simulink model "cbuildv0p5"  (R2024b)
settings: Solver=FixedStepAuto  StartTime=0.0  StopTime=12  FixedStep=0.001  RelTol=1e-3
model workspace (MAT data in the model file):
  C = 19480.5566856
  DGain = [16.29965735 16.29965735 15.46224499 15.46224499 15.85491435 21.71073697 22.54158281 11.7271646 11.89023926 12.01707508 12.11854371 12.20156349 12.27074664 12.32928621 12.37946299]
  FBgain = 1
  FFgain = 0.7
  GR = 14.14
  IGain = [117.4799242 117.4799242 87.54143949 87.54143949 65.86609231 58.19090765 57.39102046 195.6414284 195.4270634 195.2603347 195.1269515 195.0178196 194.9268763 194.8499242 194.7839652]
  Izz = 76.97
  Kb = 5
  Kd = 2
  Ki = 10
  Kn = 1
  Kp = 0.1
  L = 1.53
  Mz_to_CMD_TV_delta = 1
  NGain = [2.84450804 2.84450804 4.245826716 5.412937893 3.440885499 2 2 14.58729627 14.58729627 14.58729627 14.58729627 14.58729627 14.58729627 14.58729627 14.58729627]
  PGain = [130.03354 130.03354 132.2979663 135.8088906 130.4448578 122.5111241 121.680406 275.8117795 275.6454267 275.5160406 275.4125314 275.3278419 275.2572671 275.1975499 275.1463636]
  R_e = 0.197
  Tmax = 21
  Tmin = 0
  a = 0.775
  degrees_to_radians = 0.0174772222222
  g = 9.81
  h = 0.225
  kappa_desired = 0.2
  kph_to_m = 0.277777777778
  kph_to_mpers = 0.277777777778
  m = 278
  mu = 1
  rpm_to_radpers = 0.10472
  steering_ratio = 1.17517328292
  t = 1.2
  vx_vector = [0 3.21428571429 6.42857142857 9.64285714286 12.8571428571 16.0714285714 19.2857142857 22.5 25.7142857143 28.9285714286 32.1428571429 35.3571428571 38.5714285714 41.7857142857 45]
libraries: slpidlib x2, Solver_SF x1, simulink x1
settings Model: Creator=kara.28  LastModifiedBy=kara.28

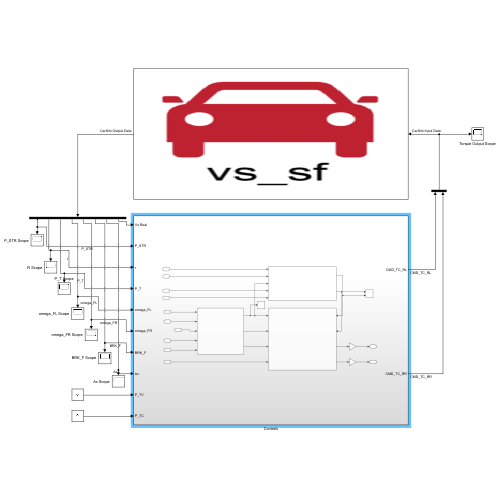
[thumbnail: Simulink's stored preview of the top-level diagram]
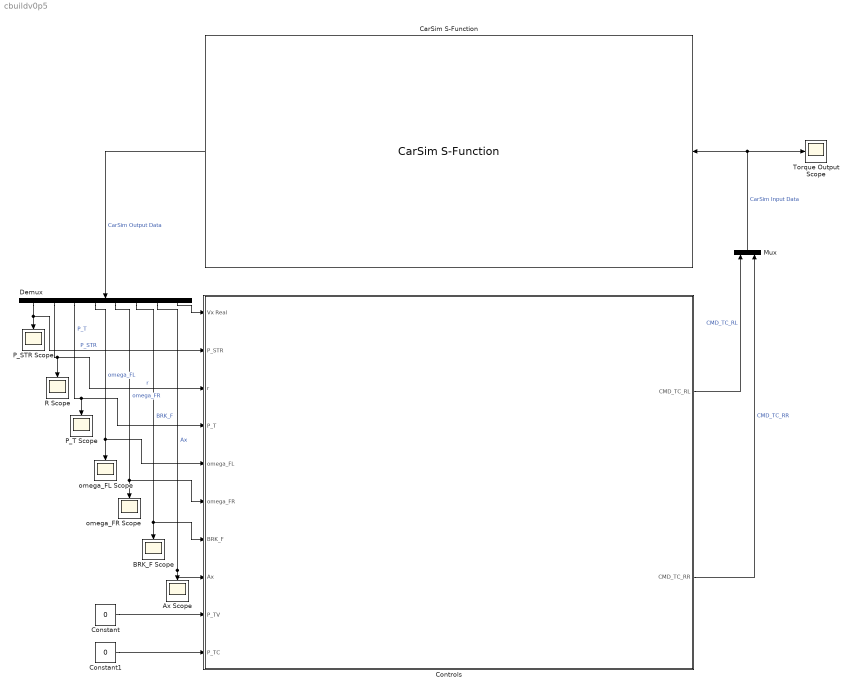
== system cbuildv0p5 ==
  Ax Scope : Scope
  BRK_F Scope : Scope
  CarSim S-Function : Solver_SF/CarSim S-Function  Priority=1  SIMFILE=simfile.sim  Run_RTs=off  vs_state_ind=Run  StopMode_ind=Vehicle Model
  Constant : Constant  Value=0
  Constant1 : Constant  Value=0
  Controls : Subsystem
  Demux : Demux  Outputs=8
  Mux : Mux  Inputs=2
  P_STR Scope : Scope
  P_T Scope : Scope
  R Scope : Scope
  Torque Output Scope : Scope
  omega_FL Scope : Scope
  omega_FR Scope : Scope
  wires:
  Constant/1 -> Controls/9(P_TV)
  Constant1/1 -> Controls/10(P_TC)
  Mux/1 -> Torque Output Scope/1, CarSim S-Function/1  "CarSim Input Data"
  CarSim S-Function/1 -> Demux/1  "CarSim Output Data"
  Demux/1 -> P_STR Scope/1, Controls/2(P_STR)  "P_STR"
  Demux/2 -> R Scope/1, Controls/3(r)  "r"
  Demux/3 -> P_T Scope/1, Controls/4(P_T)  "P_T"
  Demux/4 -> omega_FL Scope/1, Controls/5(omega_FL)  "omega_FL"
  Demux/5 -> omega_FR Scope/1, Controls/6(omega_FR)  "omega_FR"
  Demux/6 -> BRK_F Scope/1, Controls/7(BRK_F)  "BRK_F"
  Demux/7 -> Ax Scope/1, Controls/8(Ax)  "Ax"
  Controls/1(CMD_TC_RL) -> Mux/1  "CMD_TC_RL"
  Controls/2(CMD_TC_RR) -> Mux/2  "CMD_TC_RR"
  Demux/8 -> Controls/1(Vx Real)

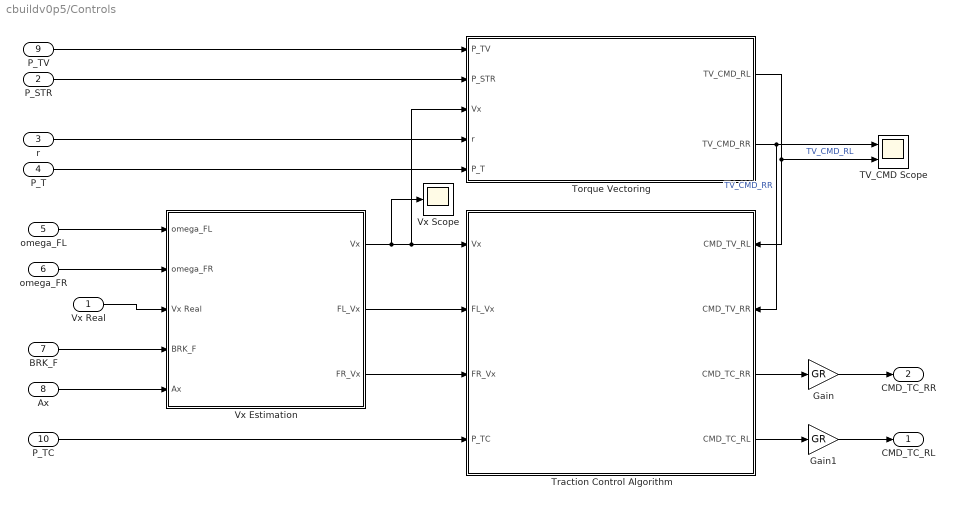
== system cbuildv0p5/Controls ==
  Vx Real : Inport
  P_STR : Inport  Port=2
  r : Inport  Port=3
  P_T : Inport  Port=4
  omega_FL : Inport  Port=5
  omega_FR : Inport  Port=6
  BRK_F : Inport  Port=7
  Ax : Inport  Port=8
  P_TV : Inport  Port=9
  P_TC : Inport  Port=10
  Gain : Gain  Gain=GR
  Gain1 : Gain  Gain=GR
  TV_CMD Scope : Scope  NumInputPorts=2
  Torque Vectoring : Subsystem
  Traction Control Algorithm : Subsystem
      settings: PortSchema="{\"entries\":[{\"content\":{\"sides\":[{\"content\":{\"connectorIds\":[\"In1\",\"In2\",\"In3\",\"In4\"]},\"type\":\"ConnectorPlacement.EquallySpacedRectSide\",\"uuid\":\"6d3224cc-3493-4876-87bf-cb750c54d205\"},{\"content\":{\"connectorIds\":[\"In5\",\"In6\",\"Out1\",\"Out2\"],\"side\":\"RIGHT\"},\"type\":\"ConnectorPlacement.EquallySpacedRectSide\",\"uuid\":\"16bb671c-e18d-4977-8b66-2f7bbb636356\"},{\"content\":{\"side\":\"TOP\"},\"type\":\"ConnectorPlacement.EquallySpacedRectSide\",\"uuid\":\"70c91239-ad82-48f3-8aa3-48d7bdfb7bbb\"}]},\"type\":\"ConnectorPlacement.EquallySpacedConnector\",\"uuid\":\"0f8ba5f7-72f2-430e-8458-63f00911aa7a\"}],\"packageUris\":[\"http://schema.mathworks.com/mf0/Connector/R2020b\"],\"version\":\"1.0\"}"
  Vx Estimation : Subsystem
  Vx Scope : Scope
  CMD_TC_RL : Outport
  CMD_TC_RR : Outport  Port=2
  wires:
  omega_FL/1 -> Vx Estimation/1(omega_FL)
  Vx Estimation/3(FR_Vx) -> Traction Control Algorithm/3(FR_Vx)
  Torque Vectoring/1(TV_CMD_RL) -> Traction Control Algorithm/5(CMD_TV_RL), TV_CMD Scope/2  "TV_CMD_RL"
  P_STR/1 -> Torque Vectoring/2(P_STR)
  Vx Estimation/2(FL_Vx) -> Traction Control Algorithm/2(FL_Vx)
  Vx Estimation/1(Vx) -> Vx Scope/1, Torque Vectoring/3(Vx), Traction Control Algorithm/1(Vx)
  P_T/1 -> Torque Vectoring/5(P_T)
  Ax/1 -> Vx Estimation/5(Ax)
  BRK_F/1 -> Vx Estimation/4(BRK_F)
  P_TC/1 -> Traction Control Algorithm/4(P_TC)
  omega_FR/1 -> Vx Estimation/2(omega_FR)
  Traction Control Algorithm/2(CMD_TC_RL) -> Gain1/1
  P_TV/1 -> Torque Vectoring/1(P_TV)
  Traction Control Algorithm/1(CMD_TC_RR) -> Gain/1
  r/1 -> Torque Vectoring/4(r)
  Torque Vectoring/2(TV_CMD_RR) -> Traction Control Algorithm/6(CMD_TV_RR), TV_CMD Scope/1  "TV_CMD_RR"
  Vx Real/1 -> Vx Estimation/3(Vx Real)
  Gain/1 -> CMD_TC_RR/1
  Gain1/1 -> CMD_TC_RL/1

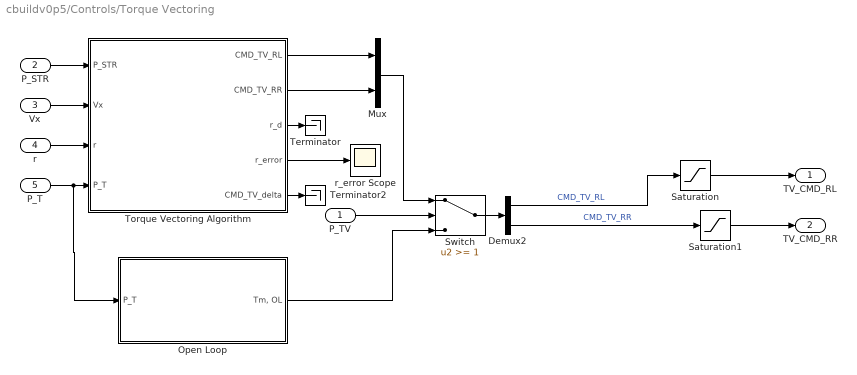
== system cbuildv0p5/Controls/Torque Vectoring ==
  P_TV : Inport
  P_STR : Inport  Port=2
  Vx : Inport  Port=3
  r : Inport  Port=4
  P_T : Inport  Port=5
  Demux2 : Demux  Outputs=2
  Mux : Mux  Inputs=2
  Open Loop : Subsystem
  Saturation : Saturate  UpperLimit=Tmax  LowerLimit=Tmin
  Saturation1 : Saturate  UpperLimit=Tmax  LowerLimit=Tmin
  Switch : Switch  Threshold=1  SaturateOnIntegerOverflow=off  InputSameDT=off
  Terminator : Terminator
  Terminator2 : Terminator
  Torque Vectoring Algorithm : Subsystem
  r_error Scope : Scope
  TV_CMD_RL : Outport
  TV_CMD_RR : Outport  Port=2
  wires:
  Demux2/2 -> Saturation1/1  "CMD_TV_RR"
  Mux/1 -> Switch/1
  P_TV/1 -> Switch/2
  Torque Vectoring Algorithm/2(CMD_TV_RR) -> Mux/2
  Demux2/1 -> Saturation/1  "CMD_TV_RL"
  Open Loop/1("Tm, OL") -> Switch/3
  Torque Vectoring Algorithm/1(CMD_TV_RL) -> Mux/1
  Switch/1 -> Demux2/1
  P_STR/1 -> Torque Vectoring Algorithm/1(P_STR)
  Vx/1 -> Torque Vectoring Algorithm/2(Vx)
  r/1 -> Torque Vectoring Algorithm/3(r)
  P_T/1 -> Open Loop/1(P_T), Torque Vectoring Algorithm/4(P_T)
  Torque Vectoring Algorithm/3(r_d) -> Terminator/1
  Torque Vectoring Algorithm/4(r_error) -> r_error Scope/1
  Torque Vectoring Algorithm/5(CMD_TV_delta) -> Terminator2/1
  Saturation/1 -> TV_CMD_RL/1
  Saturation1/1 -> TV_CMD_RR/1

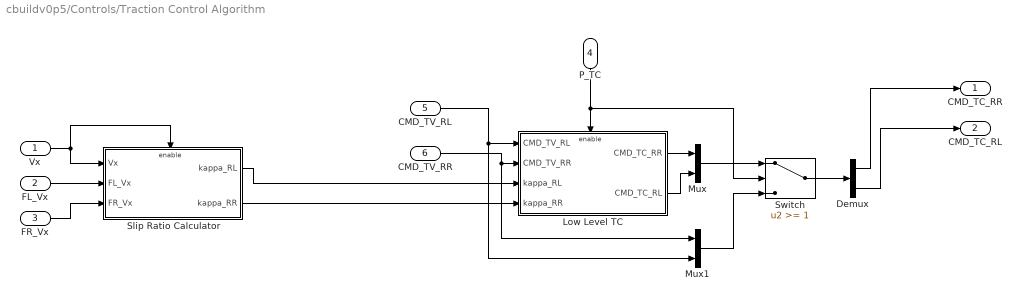
== system cbuildv0p5/Controls/Traction Control Algorithm ==
  Vx : Inport
  FL_Vx : Inport  Port=2
  FR_Vx : Inport  Port=3
  P_TC : Inport  Port=4
  CMD_TV_RL : Inport  Port=5
  CMD_TV_RR : Inport  Port=6
  Demux : Demux  Outputs=2
  Low Level TC : Subsystem
  Mux : Mux  Inputs=2
  Mux1 : Mux  Inputs=2
  Slip Ratio Calculator : Subsystem
  Switch : Switch  Threshold=1  SaturateOnIntegerOverflow=off  InputSameDT=off
  CMD_TC_RR : Outport
  CMD_TC_RL : Outport  Port=2
  wires:
  Slip Ratio Calculator/2(kappa_RR) -> Low Level TC/4(kappa_RR)
  Slip Ratio Calculator/1(kappa_RL) -> Low Level TC/3(kappa_RL)
  FL_Vx/1 -> Slip Ratio Calculator/2(FL_Vx)
  Vx/1 -> Slip Ratio Calculator/Enable, Slip Ratio Calculator/1(Vx)
  FR_Vx/1 -> Slip Ratio Calculator/3(FR_Vx)
  CMD_TV_RL/1 -> Mux1/2, Low Level TC/1(CMD_TV_RL)
  CMD_TV_RR/1 -> Mux1/1, Low Level TC/2(CMD_TV_RR)
  Low Level TC/1(CMD_TC_RR) -> Mux/1
  Low Level TC/2(CMD_TC_RL) -> Mux/2
  Mux/1 -> Switch/1
  Mux1/1 -> Switch/3
  Switch/1 -> Demux/1
  Demux/1 -> CMD_TC_RR/1
  Demux/2 -> CMD_TC_RL/1
  P_TC/1 -> Switch/2, Low Level TC/Enable

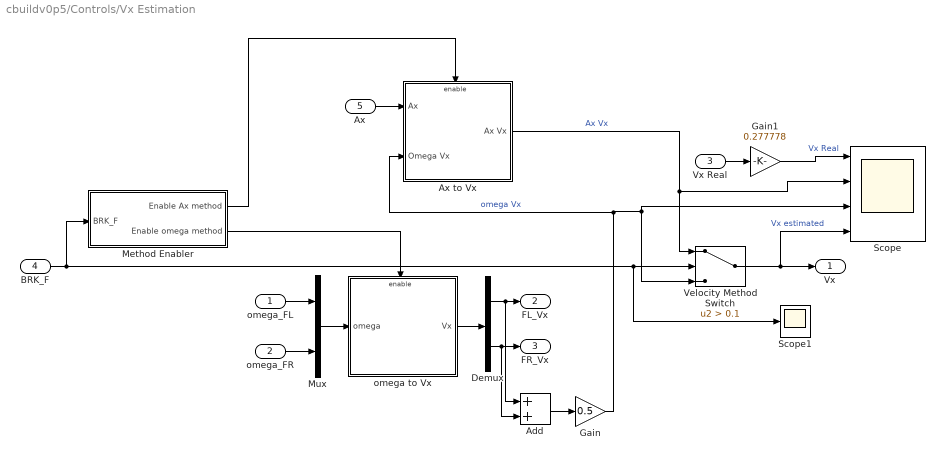
== system cbuildv0p5/Controls/Vx Estimation ==
  omega_FL : Inport
  omega_FR : Inport  Port=2
  Vx Real : Inport  Port=3
  BRK_F : Inport  Port=4
  Ax : Inport  Port=5
  Add : Sum
  Ax to Vx : Subsystem
  Demux : Demux  Outputs=2
  Gain : Gain  Gain=0.5
  Gain1 : Gain  Gain=0.277778
  Method Enabler : Subsystem
  Mux : Mux  Inputs=2
  Scope : Scope  NumInputPorts=4
  Scope1 : Scope
  Velocity Method Switch : Switch  Criteria=u2 > Threshold  Threshold=0.1  SaturateOnIntegerOverflow=off  InputSameDT=off
  omega to Vx : Subsystem
  Vx : Outport
  FL_Vx : Outport  Port=2
  FR_Vx : Outport  Port=3
  wires:
  Mux/1 -> omega to Vx/1(omega)
  omega to Vx/1(Vx) -> Demux/1
  Demux/2 -> Add/2, FR_Vx/1
  omega_FR/1 -> Mux/2
  omega_FL/1 -> Mux/1
  Demux/1 -> Add/1, FL_Vx/1
  BRK_F/1 -> Scope1/1, Velocity Method Switch/2, Method Enabler/1(BRK_F)
  Add/1 -> Gain/1
  Gain/1 -> Velocity Method Switch/3, Scope/3, Ax to Vx/2(Omega Vx)  "omega Vx"
  Velocity Method Switch/1 -> Vx/1, Scope/4  "Vx estimated"
  Ax/1 -> Ax to Vx/1(Ax)
  Ax to Vx/1(Ax Vx) -> Velocity Method Switch/1, Scope/2  "Ax Vx"
  Method Enabler/2(Enable omega method) -> omega to Vx/Enable
  Vx Real/1 -> Gain1/1
  Gain1/1 -> Scope/1  "Vx Real"
  Method Enabler/1(Enable Ax method) -> Ax to Vx/Enable

== system cbuildv0p5/Controls/Torque Vectoring/Open Loop ==
  P_T : Inport
  Gain : Gain  Gain=Tmax
  "Tm, OL" : Outport
  wires:
  P_T/1 -> Gain/1
  Gain/1 -> "Tm, OL"/1

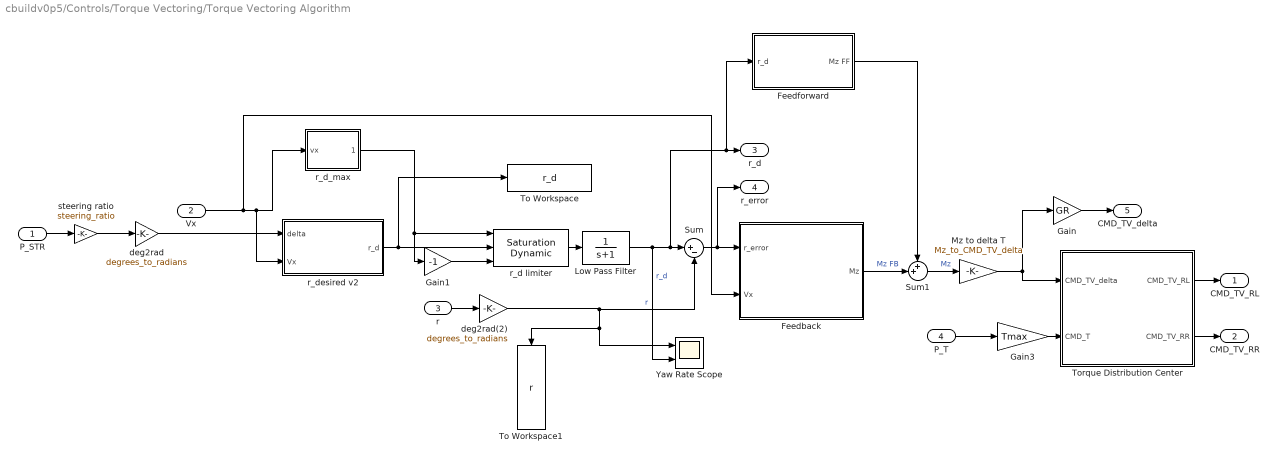
== system cbuildv0p5/Controls/Torque Vectoring/Torque Vectoring Algorithm ==
  P_STR : Inport
  Vx : Inport  Port=2
  r : Inport  Port=3
  P_T : Inport  Port=4
  Feedback : Subsystem
  Feedforward : Subsystem
  Gain : Gain  Gain=GR
  Gain1 : Gain  Gain=-1
  Gain3 : Gain  Gain=Tmax
  Low Pass Filter : TransferFcn  Denominator=[1 1]
  Mz to delta T : Gain  Gain=Mz_to_CMD_TV_delta
  Sum : Sum  Inputs=|+-
  Sum1 : Sum  Inputs=++|
  To Workspace : ToWorkspace  VariableName=r_d  SampleTime=-1
  To Workspace1 : ToWorkspace  VariableName=r  SampleTime=-1
  Torque Distribution Center : Subsystem
  Yaw Rate Scope : Scope  NumInputPorts=2
  deg2rad : Gain  Gain=degrees_to_radians
  deg2rad(2) : Gain  Gain=degrees_to_radians
  r_d limiter : simulink/Discontinuities/Saturation Dynamic  OutMin=[]  OutMax=[]  OutDataTypeStr=Inherit: Same as second input  OutDataType=fixdt(1, 16)  OutScaling=2^-10  RndMeth=Round  DoSatur=off
  r_d_max : Subsystem
  r_desired v2 : Subsystem
  steering ratio : Gain  Gain=steering_ratio
  CMD_TV_RL : Outport
  CMD_TV_RR : Outport  Port=2
  r_d : Outport  Port=3
  r_error : Outport  Port=4
  CMD_TV_delta : Outport  Port=5
  wires:
  r_d_max/1(r_d_max) -> r_d limiter/1, Gain1/1
  Sum/1 -> r_error/1, Feedback/1(r_error)
  Gain3/1 -> Torque Distribution Center/2(CMD_T)
  r/1 -> deg2rad(2)/1
  Gain1/1 -> r_d limiter/3
  P_T/1 -> Gain3/1
  Mz to delta T/1 -> Gain/1, Torque Distribution Center/1(CMD_TV_delta)
  deg2rad/1 -> r_desired v2/1(delta)
  Vx/1 -> Feedback/2(Vx), r_desired v2/2(Vx), r_d_max/1(vx)
  Feedback/1(Mz) -> Sum1/2  "Mz FB"
  Sum1/1 -> Mz to delta T/1  "Mz"
  r_d limiter/1 -> Low Pass Filter/1
  Low Pass Filter/1 -> Yaw Rate Scope/2, Sum/1, Feedforward/1(r_d), r_d/1  "r_d"
  Feedforward/1(Mz FF) -> Sum1/1
  Torque Distribution Center/1(CMD_TV_RL) -> CMD_TV_RL/1
  Torque Distribution Center/2(CMD_TV_RR) -> CMD_TV_RR/1
  Gain/1 -> CMD_TV_delta/1
  P_STR/1 -> steering ratio/1
  steering ratio/1 -> deg2rad/1
  r_desired v2/1(r_d) -> To Workspace/1, r_d limiter/2
  deg2rad(2)/1 -> Sum/2, Yaw Rate Scope/1, To Workspace1/1  "r"

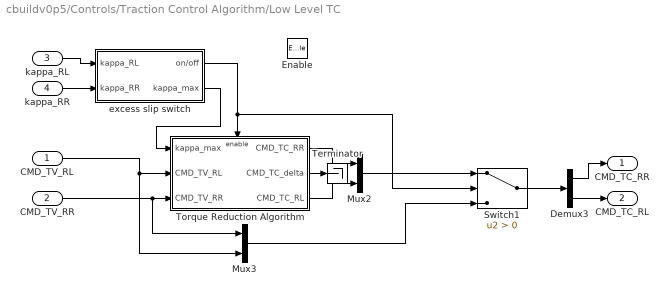
== system cbuildv0p5/Controls/Traction Control Algorithm/Low Level TC ==
  CMD_TV_RL : Inport
  CMD_TV_RR : Inport  Port=2
  kappa_RL : Inport  Port=3
  kappa_RR : Inport  Port=4
  Enable : EnablePort
  Demux3 : Demux  Outputs=2
  Mux2 : Mux  Inputs=2
  Mux3 : Mux  Inputs=2
  Switch1 : Switch  Criteria=u2 > Threshold  SaturateOnIntegerOverflow=off  InputSameDT=off
  Terminator : Terminator
  Torque Reduction Algorithm : Subsystem  TreatAsAtomicUnit=on
  excess slip switch : Subsystem
  CMD_TC_RR : Outport
  CMD_TC_RL : Outport  Port=2
  wires:
  Demux3/2 -> CMD_TC_RL/1
  Mux3/1 -> Switch1/3
  CMD_TV_RL/1 -> Mux3/2, Torque Reduction Algorithm/2(CMD_TV_RL)
  Torque Reduction Algorithm/2(CMD_TC_delta) -> Terminator/1
  CMD_TV_RR/1 -> Mux3/1, Torque Reduction Algorithm/3(CMD_TV_RR)
  Torque Reduction Algorithm/1(CMD_TC_RR) -> Mux2/1
  excess slip switch/1(on/off) -> Switch1/2, Torque Reduction Algorithm/Enable
  Mux2/1 -> Switch1/1
  Torque Reduction Algorithm/3(CMD_TC_RL) -> Mux2/2
  Switch1/1 -> Demux3/1
  Demux3/1 -> CMD_TC_RR/1
  excess slip switch/2(kappa_max) -> Torque Reduction Algorithm/1(kappa_max)
  kappa_RL/1 -> excess slip switch/1(kappa_RL)
  kappa_RR/1 -> excess slip switch/2(kappa_RR)

== system cbuildv0p5/Controls/Traction Control Algorithm/Slip Ratio Calculator ==
  Vx : Inport
  FL_Vx : Inport  Port=2
  FR_Vx : Inport  Port=3
  Enable : EnablePort
  Divide : Product  Inputs=*/
  Divide1 : Product  Inputs=*/
  Scope : Scope  NumInputPorts=2
  Subtract : Sum  Inputs=+-
  Subtract1 : Sum  Inputs=+-
  kappa_RL : Outport
  kappa_RR : Outport  Port=2
  wires:
  Subtract/1 -> Divide/1
  Vx/1 -> Subtract1/1, Divide/2, Divide1/2, Subtract/1
  Divide/1 -> Scope/1, kappa_RL/1
  Subtract1/1 -> Divide1/1
  FL_Vx/1 -> Subtract/2
  FR_Vx/1 -> Subtract1/2
  Divide1/1 -> kappa_RR/1, Scope/2

== system cbuildv0p5/Controls/Vx Estimation/Ax to Vx ==
  Ax : Inport
  Omega Vx : Inport  Port=2
  Enable : EnablePort
  Integrator : Integrator
  Plus : Sum
  to m/s^2 : Gain  Gain=g
  Ax Vx : Outport
  wires:
  Ax/1 -> to m/s^2/1
  Integrator/1 -> Plus/2
  Omega Vx/1 -> Plus/1
  Plus/1 -> Ax Vx/1
  to m/s^2/1 -> Integrator/1

== system cbuildv0p5/Controls/Vx Estimation/Method Enabler ==
  BRK_F : Inport
  Constant : Constant  Value=0
  Constant1 : Constant
  Constant2 : Constant  Value=0
  Constant3 : Constant
  Switch : Switch  Criteria=u2 > Threshold  Threshold=0.1  SaturateOnIntegerOverflow=off  InputSameDT=off
  Switch1 : Switch  Criteria=u2 > Threshold  SaturateOnIntegerOverflow=off  InputSameDT=off
  Enable Ax method : Outport
  Enable omega method : Outport  Port=2
  wires:
  Constant1/1 -> Switch/3
  Constant/1 -> Switch/1
  BRK_F/1 -> Switch/2
  Constant2/1 -> Switch1/1
  Constant3/1 -> Switch1/3
  Switch1/1 -> Enable Ax method/1
  Switch/1 -> Enable omega method/1, Switch1/2

== system cbuildv0p5/Controls/Vx Estimation/omega to Vx ==
  omega : Inport
  Enable : EnablePort
  Gain : Gain  Gain=R_e
  Gain1 : Gain  Gain=rpm_to_radpers
  Vx : Outport
  wires:
  omega/1 -> Gain1/1
  Gain/1 -> Vx/1
  Gain1/1 -> Gain/1

== system cbuildv0p5/Controls/Torque Vectoring/Torque Vectoring Algorithm/Feedback ==
  r_error : Inport
  Vx : Inport  Port=2
  D Gains : Lookup_n-D  NumberOfTableDimensions=1  LookupTableObject=''  BreakpointsForDimension1=vx_vector  BreakpointsForDimension1FirstPoint=10  BreakpointsForDimension2FirstPoint=10  BreakpointsForDimension1Spacing=12  BreakpointsForDimension2Spacing=12  IndexSearchMethod=Evenly spaced points  Table=DGain  RemoveProtectionInput=on  InternalRulePriority=Speed  RndMeth=Simplest
  Gain : Gain  Gain=FBgain
  Gain1 : Gain  Gain=Kp
  Gain2 : Gain  Gain=Ki
  Gain3 : Gain  Gain=Kd
  Gain4 : Gain  Gain=Kn
  I Gains : Lookup_n-D  NumberOfTableDimensions=1  LookupTableObject=''  BreakpointsForDimension1=vx_vector  BreakpointsForDimension1FirstPoint=10  BreakpointsForDimension2FirstPoint=10  BreakpointsForDimension1Spacing=12  BreakpointsForDimension2Spacing=12  IndexSearchMethod=Evenly spaced points  Table=IGain  RemoveProtectionInput=on  InternalRulePriority=Speed  RndMeth=Simplest
  N Gains : Lookup_n-D  NumberOfTableDimensions=1  LookupTableObject=''  BreakpointsForDimension1=vx_vector  BreakpointsForDimension1FirstPoint=10  BreakpointsForDimension2FirstPoint=10  BreakpointsForDimension1Spacing=12  BreakpointsForDimension2Spacing=12  IndexSearchMethod=Evenly spaced points  Table=NGain  RemoveProtectionInput=on  InternalRulePriority=Speed  RndMeth=Simplest
  P Gains : Lookup_n-D  NumberOfTableDimensions=1  LookupTableObject=''  BreakpointsForDimension1=vx_vector  BreakpointsForDimension1FirstPoint=10  BreakpointsForDimension2FirstPoint=10  BreakpointsForDimension1Spacing=12  BreakpointsForDimension2Spacing=12  IndexSearchMethod=Evenly spaced points  Table=PGain  RemoveProtectionInput=on  InternalRulePriority=Speed  RndMeth=Simplest
  PID Controller : slpidlib/PID Controller  Controller=PID  Form=Parallel  TimeDomain=Continuous-time  UseExternalTs=off  SampleTime=-1  IntegratorMethod=Forward Euler  FilterMethod=Forward Euler  ControllerParametersSource=external  P=122.511124072632  I=58.1909076470783  UseKiTs=off  D=21.7107369694367  UseExternalDerivativeSource=off  N=2  UseFilter=on  TunerSelectOption=Transfer Function Based (PID Tuner App)  InitialConditionSource=internal  InitialConditionForIntegrator=0  InitialConditionForFilter=0  DifferentiatorICPrevScaledInput=0  ExternalReset=none  TrackingMode=off  Kt=1  LimitOutput=on  SatLimitsSource=internal  UpperSaturationLimit=10  LowerSaturationLimit=-10  LinearizeAsGain=on  AntiWindupMode=back-calculation  Kb=Kb  LimitIntegrator=off  UpperIntegratorSaturationLimit=inf  LowerIntegratorSaturationLimit=-inf  POutMin=[]  POutMax=[]  IOutMin=[]  IOutMax=[]  DOutMin=[]  DOutMax=[]  NOutMin=[]  NOutMax=[]  SumOutMin=[]  SumOutMax=[]  SaturationOutMin=[]  SaturationOutMax=[]  PParamMin=[]  PParamMax=[]  IParamMin=[]  IParamMax=[]  DParamMin=[]  DParamMax=[]  NParamMin=[]  NParamMax=[]  KbParamMin=[]  KbParamMax=[]  KtParamMin=[]  KtParamMax=[]  KbOutMin=[]  KbOutMax=[]  KtOutMin=[]  KtOutMax=[]  IntegratorOutMin=[]  IntegratorOutMax=[]  FilterOutMin=[]  FilterOutMax=[]  SumI1OutMin=[]  SumI1OutMax=[]  SumI2OutMin=[]  SumI2OutMax=[]  SumI3OutMin=[]  SumI3OutMax=[]  SumI4OutMin=[]  SumI4OutMax=[]  SumDOutMin=[]  SumDOutMax=[]  DifferentiatorOutMin=[]  DifferentiatorOutMax=[]  FilterDiffOutCoefMin=[]  FilterDiffOutCoefMax=[]  ReciprocalOutMin=[]  ReciprocalOutMax=[]  SumDenOutMin=[]  SumDenOutMax=[]  SumNumOutMin=[]  SumNumOutMax=[]  DivideOutMin=[]  DivideOutMax=[]  UdiffTsProdOutMin=[]  UdiffTsProdOutMax=[]  NTsProdOutMin=[]  NTsProdOutMax=[]  UintegralTsProdOutMin=[]  UintegralTsProdOutMax=[]  UngainTsProdOutMin=[]  UngainTsProdOutMax=[]  ClampingZeroOutDataTypeStr=Inherit: Inherit via back propagation  ClampingZeroOutMin=[]  ClampingZeroOutMax=[]  FilterDenConstantOutDataTypeStr=Inherit: Inherit via back propagation  FilterDenConstantOutMin=[]  FilterDenConstantOutMax=[]  PCopyOutDataTypeStr=Inherit: Inherit via back propagation  PCopyOutMin=[]  PCopyOutMax=[]  NCopyOutDataTypeStr=Inherit: Inherit via back propagation  NCopyOutMin=[]  NCopyOutMax=[]  IntegratorContinuousStateAttributes=''  IntegratorStateMustResolveToSignalObject=off  IntegratorRTWStateStorageClass=Auto  FilterContinuousStateAttributes=''  FilterStateMustResolveToSignalObject=off  FilterRTWStateStorageClass=Auto  ParallelPVariant=ExternalParameters  IdealPVariant=Disabled  IVariant=ExternalParameters  DVariant=ExternalParameters  IntegratorVariant=Continuous  SatVariant=Enabled  AWVariant=BackCalculation  PCopyVariant=Disabled  TRVariant=Disabled  FdbkBlocksVariant=Forward  IdealPFdbkVariant=Disabled  SatFdbkVariant=Disabled  DerivativeFilterVariant=ContFilter  NVariant=ExternalParameters  NCopyVariant=Disabled  FilterICVariant=InternalICsFilter  IntegratorICVariant=InternalICs  ExternalResetVariant=Disabled  TRSumVariant=Passthrough  SumFdbkVariant=Disabled  SumVariant=Sum_PID  TsampFilterVariant=InternalTs  TsampNgainVariant=Passthrough  TsampIntegralVariant=Disabled_SignalSpec  ExternalSaturationOutDataTypeStr=Inherit: Same as second input  DerivativeSourceVariant=ErrorSignal  PreIntVariant=InternalPreInt
  Mz : Outport
  wires:
  r_error/1 -> PID Controller/1
  Vx/1 -> N Gains/1, D Gains/1, I Gains/1, P Gains/1
  I Gains/1 -> Gain2/1
  N Gains/1 -> Gain4/1
  PID Controller/1 -> Gain/1
  Gain/1 -> Mz/1
  P Gains/1 -> Gain1/1
  D Gains/1 -> Gain3/1
  Gain1/1 -> PID Controller/2
  Gain2/1 -> PID Controller/3
  Gain3/1 -> PID Controller/4
  Gain4/1 -> PID Controller/5

== system cbuildv0p5/Controls/Torque Vectoring/Torque Vectoring Algorithm/Feedforward ==
  r_d : Inport
  Gain : Gain  Gain=Izz
  Gain2 : Gain  Gain=FFgain
  Mz FF : Outport
  wires:
  r_d/1 -> Gain/1
  Gain/1 -> Gain2/1
  Gain2/1 -> Mz FF/1  "Mz FF"

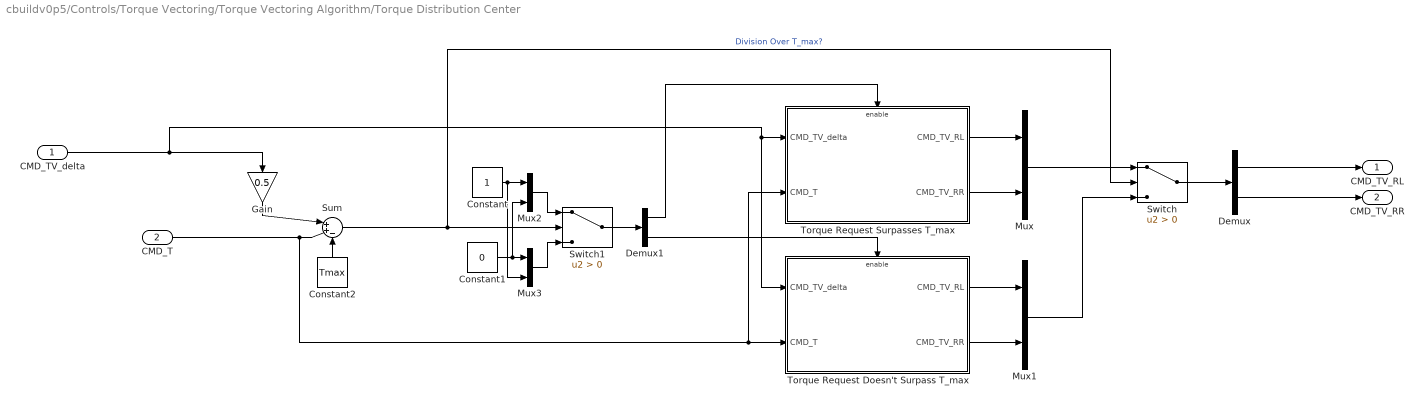
== system cbuildv0p5/Controls/Torque Vectoring/Torque Vectoring Algorithm/Torque Distribution Center ==
  CMD_TV_delta : Inport
  CMD_T : Inport  Port=2
  Constant : Constant
  Constant1 : Constant  Value=0
  Constant2 : Constant  Value=Tmax
  Demux : Demux  Outputs=2
  Demux1 : Demux  Outputs=2
  Gain : Gain  Gain=0.5
  Mux{,1..3} (4 alike) : Mux  Inputs=2
  Sum : Sum  Inputs=|++-
  Switch : Switch  Criteria=u2 > Threshold  SaturateOnIntegerOverflow=off  InputSameDT=off
  Switch1 : Switch  Criteria=u2 > Threshold  SaturateOnIntegerOverflow=off  InputSameDT=off
  Torque Request Doesn't Surpass T_max : Subsystem  TreatAsAtomicUnit=on
  Torque Request Surpasses T_max : Subsystem  TreatAsAtomicUnit=on
  CMD_TV_RL : Outport
  CMD_TV_RR : Outport  Port=2
  wires:
  Sum/1 -> Switch1/2, Switch/2  "Division Over T_max?"
  Gain/1 -> Sum/1
  CMD_TV_delta/1 -> Gain/1, Torque Request Doesn't Surpass T_max/1(CMD_TV_delta), Torque Request Surpasses T_max/1(CMD_TV_delta)
  Torque Request Surpasses T_max/1(CMD_TV_RL) -> Mux/1
  Torque Request Surpasses T_max/2(CMD_TV_RR) -> Mux/2
  Torque Request Doesn't Surpass T_max/1(CMD_TV_RL) -> Mux1/1
  Torque Request Doesn't Surpass T_max/2(CMD_TV_RR) -> Mux1/2
  Mux/1 -> Switch/1
  Mux1/1 -> Switch/3
  Switch/1 -> Demux/1
  CMD_T/1 -> Torque Request Surpasses T_max/2(CMD_T), Torque Request Doesn't Surpass T_max/2(CMD_T), Sum/2
  Mux2/1 -> Switch1/1
  Mux3/1 -> Switch1/3
  Switch1/1 -> Demux1/1
  Demux1/1 -> Torque Request Surpasses T_max/Enable
  Demux1/2 -> Torque Request Doesn't Surpass T_max/Enable
  Constant/1 -> Mux2/1, Mux3/2
  Constant1/1 -> Mux2/2, Mux3/1
  Demux/1 -> CMD_TV_RL/1
  Demux/2 -> CMD_TV_RR/1
  Constant2/1 -> Sum/3

== system cbuildv0p5/Controls/Torque Vectoring/Torque Vectoring Algorithm/r_d_max ==
  vx : Inport
  Constant : Constant  Value=0.85*mu*g/(1+(h/t))
  Divide : Product  Inputs=*/
  Saturation : Saturate  UpperLimit=1000000  LowerLimit=0.01
  r_d_max : Outport
  wires:
  Constant/1 -> Divide/1
  vx/1 -> Saturation/1
  Saturation/1 -> Divide/2
  Divide/1 -> r_d_max/1

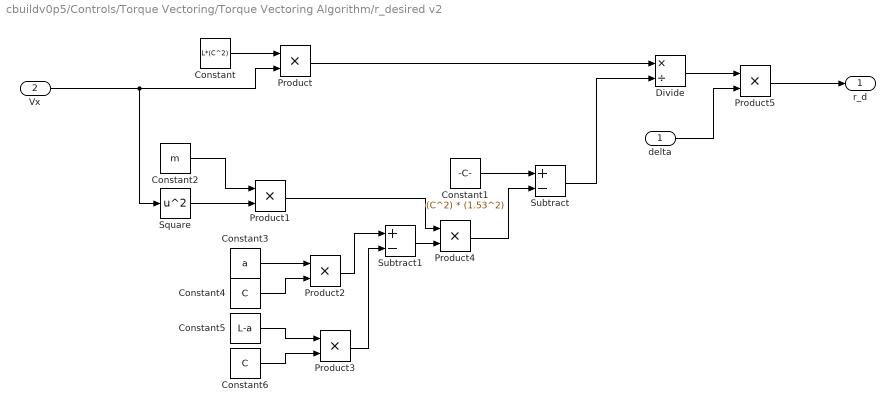
== system cbuildv0p5/Controls/Torque Vectoring/Torque Vectoring Algorithm/r_desired v2 ==
  delta : Inport
  Vx : Inport  Port=2
  Constant : Constant  Value=L*(C^2)
  Constant1 : Constant  Value=(C^2) * (1.53^2)
  Constant2 : Constant  Value=m
  Constant3 : Constant  Value=a
  Constant4 : Constant  Value=C
  Constant5 : Constant  Value=L-a
  Constant6 : Constant  Value=C
  Divide : Product  Inputs=*/
  Product{,1..5} (6 alike) : Product
  Square : Math  Operator=square
  Subtract : Sum  Inputs=+-
  Subtract1 : Sum  Inputs=+-
  r_d : Outport
  wires:
  Constant/1 -> Product/1
  Constant1/1 -> Subtract/1
  Square/1 -> Product1/2
  Constant2/1 -> Product1/1
  Product2/1 -> Subtract1/1
  Product3/1 -> Subtract1/2
  Subtract1/1 -> Product4/2
  Product1/1 -> Product4/1
  delta/1 -> Product5/2
  Constant5/1 -> Product3/1
  Constant6/1 -> Product3/2
  Constant3/1 -> Product2/1
  Constant4/1 -> Product2/2
  Product4/1 -> Subtract/2
  Divide/1 -> Product5/1
  Product/1 -> Divide/1
  Subtract/1 -> Divide/2
  Product5/1 -> r_d/1
  Vx/1 -> Square/1, Product/2

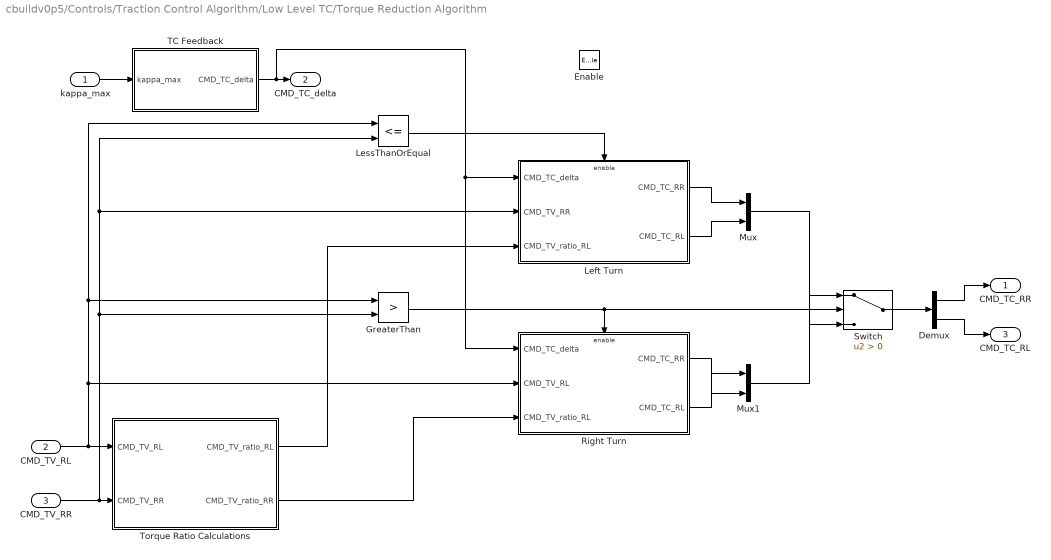
== system cbuildv0p5/Controls/Traction Control Algorithm/Low Level TC/Torque Reduction Algorithm ==
  kappa_max : Inport
  CMD_TV_RL : Inport  Port=2
  CMD_TV_RR : Inport  Port=3
  Enable : EnablePort
  Demux : Demux  Outputs=2
  GreaterThan : RelationalOperator  Operator=>  OutDataTypeStr=boolean  RndMeth=Simplest  InputSameDT=off
  Left Turn : Subsystem  TreatAsAtomicUnit=on
  LessThanOrEqual : RelationalOperator  Operator=<=  OutDataTypeStr=boolean  RndMeth=Simplest  InputSameDT=off
  Mux : Mux  Inputs=2
  Mux1 : Mux  Inputs=2
  Right Turn : Subsystem  TreatAsAtomicUnit=on
  Switch : Switch  Criteria=u2 > Threshold  SaturateOnIntegerOverflow=off  InputSameDT=off
  TC Feedback : Subsystem
  Torque Ratio Calculations : Subsystem
  CMD_TC_RR : Outport
  CMD_TC_delta : Outport  Port=2
  CMD_TC_RL : Outport  Port=3
  wires:
  CMD_TV_RL/1 -> GreaterThan/1, LessThanOrEqual/1, Right Turn/2(CMD_TV_RL), Torque Ratio Calculations/1(CMD_TV_RL)
  CMD_TV_RR/1 -> GreaterThan/2, LessThanOrEqual/2, Left Turn/2(CMD_TV_RR), Torque Ratio Calculations/2(CMD_TV_RR)
  LessThanOrEqual/1 -> Left Turn/Enable
  GreaterThan/1 -> Switch/2, Right Turn/Enable
  kappa_max/1 -> TC Feedback/1(kappa_max)
  TC Feedback/1(CMD_TC_delta) -> Right Turn/1(CMD_TC_delta), Left Turn/1(CMD_TC_delta), CMD_TC_delta/1
  Torque Ratio Calculations/1(CMD_TV_ratio_RL) -> Left Turn/3(CMD_TV_ratio_RL)
  Torque Ratio Calculations/2(CMD_TV_ratio_RR) -> Right Turn/3(CMD_TV_ratio_RL)
  Left Turn/1(CMD_TC_RR) -> Mux/1
  Left Turn/2(CMD_TC_RL) -> Mux/2
  Right Turn/2(CMD_TC_RL) -> Mux1/1
  Right Turn/1(CMD_TC_RR) -> Mux1/2
  Mux/1 -> Switch/3
  Mux1/1 -> Switch/1
  Switch/1 -> Demux/1
  Demux/1 -> CMD_TC_RR/1
  Demux/2 -> CMD_TC_RL/1

== system cbuildv0p5/Controls/Traction Control Algorithm/Low Level TC/excess slip switch ==
  kappa_RL : Inport
  kappa_RR : Inport  Port=2
  Constant : Constant
  Constant2 : Constant  Value=0
  Max : MinMax  Function=max  Inputs=2
  Switch1 : Switch  Criteria=u2 > Threshold  Threshold=kappa_desired  SaturateOnIntegerOverflow=off  InputSameDT=off
  on/off : Outport
  kappa_max : Outport  Port=2
  wires:
  kappa_RL/1 -> Max/1
  kappa_RR/1 -> Max/2
  Switch1/1 -> on/off/1
  Constant2/1 -> Switch1/3
  Constant/1 -> Switch1/1
  Max/1 -> Switch1/2, kappa_max/1

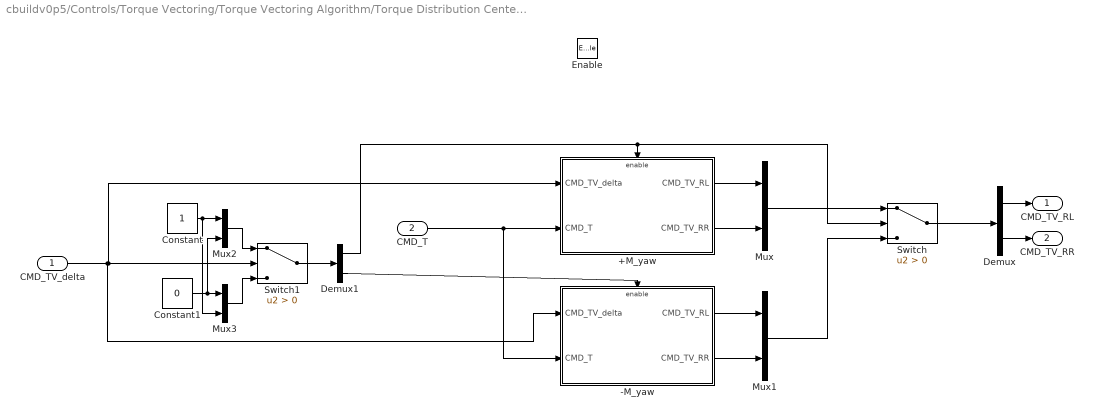
== system cbuildv0p5/Controls/Torque Vectoring/Torque Vectoring Algorithm/Torque Distribution Center/Torque Request Doesn't Surpass T_max ==
  CMD_TV_delta : Inport
  CMD_T : Inport  Port=2
  Enable : EnablePort  StatesWhenEnabling=reset
  +M_yaw : Subsystem  TreatAsAtomicUnit=on
  -M_yaw : Subsystem  TreatAsAtomicUnit=on
  Constant : Constant
  Constant1 : Constant  Value=0
  Demux : Demux  Outputs=2
  Demux1 : Demux  Outputs=2
  Mux{,1..3} (4 alike) : Mux  Inputs=2
  Switch : Switch  Criteria=u2 > Threshold  SaturateOnIntegerOverflow=off  InputSameDT=off
  Switch1 : Switch  Criteria=u2 > Threshold  SaturateOnIntegerOverflow=off  InputSameDT=off
  CMD_TV_RL : Outport
  CMD_TV_RR : Outport  Port=2
  wires:
  +M_yaw/1(CMD_TV_RL) -> Mux/1
  +M_yaw/2(CMD_TV_RR) -> Mux/2
  -M_yaw/1(CMD_TV_RL) -> Mux1/1
  -M_yaw/2(CMD_TV_RR) -> Mux1/2
  Mux/1 -> Switch/1
  Mux1/1 -> Switch/3
  CMD_T/1 -> -M_yaw/2(CMD_T), +M_yaw/2(CMD_T)
  Switch/1 -> Demux/1
  Demux/1 -> CMD_TV_RL/1
  Demux/2 -> CMD_TV_RR/1
  Mux2/1 -> Switch1/1
  Demux1/1 -> Switch/2, +M_yaw/Enable
  Demux1/2 -> -M_yaw/Enable
  Mux3/1 -> Switch1/3
  Switch1/1 -> Demux1/1
  Constant1/1 -> Mux2/2, Mux3/1
  Constant/1 -> Mux2/1, Mux3/2
  CMD_TV_delta/1 -> Switch1/2, +M_yaw/1(CMD_TV_delta), -M_yaw/1(CMD_TV_delta)

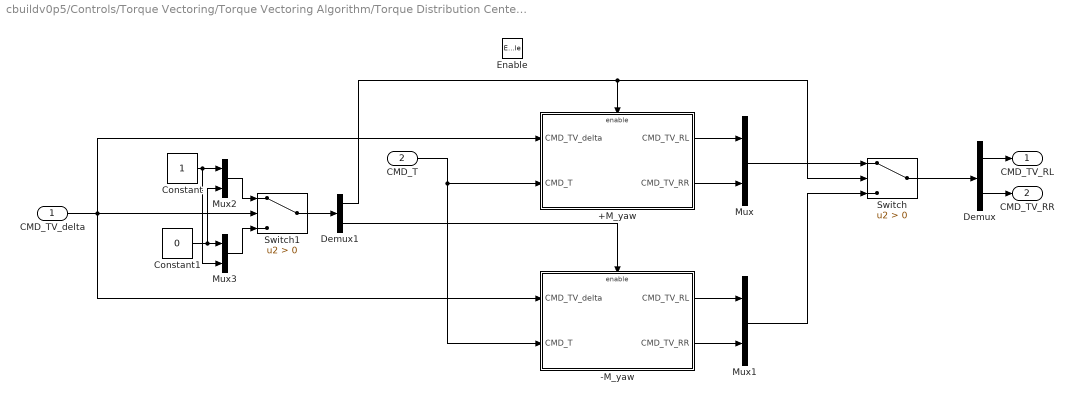
== system cbuildv0p5/Controls/Torque Vectoring/Torque Vectoring Algorithm/Torque Distribution Center/Torque Request Surpasses T_max ==
  CMD_TV_delta : Inport
  CMD_T : Inport  Port=2
  Enable : EnablePort  StatesWhenEnabling=reset
  +M_yaw : Subsystem  TreatAsAtomicUnit=on
  -M_yaw : Subsystem  TreatAsAtomicUnit=on
  Constant : Constant
  Constant1 : Constant  Value=0
  Demux : Demux  Outputs=2
  Demux1 : Demux  Outputs=2
  Mux{,1..3} (4 alike) : Mux  Inputs=2
  Switch : Switch  Criteria=u2 > Threshold  SaturateOnIntegerOverflow=off  InputSameDT=off
  Switch1 : Switch  Criteria=u2 > Threshold  SaturateOnIntegerOverflow=off  InputSameDT=off
  CMD_TV_RL : Outport
  CMD_TV_RR : Outport  Port=2
  wires:
  Mux/1 -> Switch/1
  Mux1/1 -> Switch/3
  CMD_T/1 -> -M_yaw/2(CMD_T), +M_yaw/2(CMD_T)
  Demux/2 -> CMD_TV_RR/1
  Demux/1 -> CMD_TV_RL/1
  +M_yaw/2(CMD_TV_RR) -> Mux/2
  +M_yaw/1(CMD_TV_RL) -> Mux/1
  -M_yaw/2(CMD_TV_RR) -> Mux1/2
  Switch/1 -> Demux/1
  -M_yaw/1(CMD_TV_RL) -> Mux1/1
  Mux2/1 -> Switch1/1
  Demux1/1 -> +M_yaw/Enable, Switch/2
  Demux1/2 -> -M_yaw/Enable
  Mux3/1 -> Switch1/3
  Switch1/1 -> Demux1/1
  Constant1/1 -> Mux2/2, Mux3/1
  Constant/1 -> Mux2/1, Mux3/2
  CMD_TV_delta/1 -> Switch1/2, -M_yaw/1(CMD_TV_delta), +M_yaw/1(CMD_TV_delta)

== system cbuildv0p5/Controls/Traction Control Algorithm/Low Level TC/Torque Reduction Algorithm/Left Turn ==
  CMD_TC_delta : Inport
  CMD_TV_RR : Inport  Port=2
  CMD_TV_ratio_RL : Inport  Port=3
  Enable : EnablePort
  Constant : Constant
  Divide : Product  Inputs=*/
  Saturation : Saturate  UpperLimit=inf  LowerLimit=0.001
  Subtract : Sum  Inputs=+-
  Sum : Sum  Inputs=|+-
  CMD_TC_RR : Outport
  CMD_TC_RL : Outport  Port=2
  wires:
  CMD_TV_RR/1 -> Sum/1
  CMD_TC_delta/1 -> Sum/2
  Constant/1 -> Subtract/1
  CMD_TV_ratio_RL/1 -> Subtract/2
  Sum/1 -> Divide/1, CMD_TC_RR/1
  Subtract/1 -> Saturation/1
  Saturation/1 -> Divide/2
  Divide/1 -> CMD_TC_RL/1

== system cbuildv0p5/Controls/Traction Control Algorithm/Low Level TC/Torque Reduction Algorithm/Right Turn ==
  CMD_TC_delta : Inport
  CMD_TV_RL : Inport  Port=2
  CMD_TV_ratio_RL : Inport  Port=3
  Enable : EnablePort
  Constant : Constant
  Divide : Product  Inputs=*/
  Saturation : Saturate  UpperLimit=inf  LowerLimit=0.001
  Subtract : Sum  Inputs=+-
  Sum : Sum  Inputs=|+-
  CMD_TC_RR : Outport
  CMD_TC_RL : Outport  Port=2
  wires:
  Sum/1 -> Divide/1, CMD_TC_RL/1
  CMD_TC_delta/1 -> Sum/2
  CMD_TV_ratio_RL/1 -> Subtract/2
  Saturation/1 -> Divide/2
  Constant/1 -> Subtract/1
  Subtract/1 -> Saturation/1
  Divide/1 -> CMD_TC_RR/1
  CMD_TV_RL/1 -> Sum/1

== system cbuildv0p5/Controls/Traction Control Algorithm/Low Level TC/Torque Reduction Algorithm/TC Feedback ==
  kappa_max : Inport
  Constant : Constant  Value=kappa_desired
  PID Controller : slpidlib/PID Controller  Controller=PID  Form=Parallel  TimeDomain=Continuous-time  UseExternalTs=off  SampleTime=-1  IntegratorMethod=Forward Euler  FilterMethod=Forward Euler  ControllerParametersSource=internal  P=1  I=1  UseKiTs=off  D=0  UseExternalDerivativeSource=off  N=100  UseFilter=on  TunerSelectOption=Transfer Function Based (PID Tuner App)  InitialConditionSource=internal  InitialConditionForIntegrator=0  InitialConditionForFilter=0  DifferentiatorICPrevScaledInput=0  ExternalReset=none  TrackingMode=off  Kt=1  LimitOutput=off  SatLimitsSource=internal  UpperSaturationLimit=inf  LowerSaturationLimit=-inf  LinearizeAsGain=on  AntiWindupMode=none  Kb=1  LimitIntegrator=off  UpperIntegratorSaturationLimit=inf  LowerIntegratorSaturationLimit=-inf  POutMin=[]  POutMax=[]  IOutMin=[]  IOutMax=[]  DOutMin=[]  DOutMax=[]  NOutMin=[]  NOutMax=[]  SumOutMin=[]  SumOutMax=[]  SaturationOutMin=[]  SaturationOutMax=[]  PParamMin=[]  PParamMax=[]  IParamMin=[]  IParamMax=[]  DParamMin=[]  DParamMax=[]  NParamMin=[]  NParamMax=[]  KbParamMin=[]  KbParamMax=[]  KtParamMin=[]  KtParamMax=[]  KbOutMin=[]  KbOutMax=[]  KtOutMin=[]  KtOutMax=[]  IntegratorOutMin=[]  IntegratorOutMax=[]  FilterOutMin=[]  FilterOutMax=[]  SumI1OutMin=[]  SumI1OutMax=[]  SumI2OutMin=[]  SumI2OutMax=[]  SumI3OutMin=[]  SumI3OutMax=[]  SumI4OutMin=[]  SumI4OutMax=[]  SumDOutMin=[]  SumDOutMax=[]  DifferentiatorOutMin=[]  DifferentiatorOutMax=[]  FilterDiffOutCoefMin=[]  FilterDiffOutCoefMax=[]  ReciprocalOutMin=[]  ReciprocalOutMax=[]  SumDenOutMin=[]  SumDenOutMax=[]  SumNumOutMin=[]  SumNumOutMax=[]  DivideOutMin=[]  DivideOutMax=[]  UdiffTsProdOutMin=[]  UdiffTsProdOutMax=[]  NTsProdOutMin=[]  NTsProdOutMax=[]  UintegralTsProdOutMin=[]  UintegralTsProdOutMax=[]  UngainTsProdOutMin=[]  UngainTsProdOutMax=[]  ClampingZeroOutDataTypeStr=Inherit: Inherit via back propagation  ClampingZeroOutMin=[]  ClampingZeroOutMax=[]  FilterDenConstantOutDataTypeStr=Inherit: Inherit via back propagation  FilterDenConstantOutMin=[]  FilterDenConstantOutMax=[]  PCopyOutDataTypeStr=Inherit: Inherit via back propagation  PCopyOutMin=[]  PCopyOutMax=[]  NCopyOutDataTypeStr=Inherit: Inherit via back propagation  NCopyOutMin=[]  NCopyOutMax=[]  IntegratorContinuousStateAttributes=''  IntegratorStateMustResolveToSignalObject=off  IntegratorRTWStateStorageClass=Auto  FilterContinuousStateAttributes=''  FilterStateMustResolveToSignalObject=off  FilterRTWStateStorageClass=Auto  ParallelPVariant=InternalParameters  IdealPVariant=Disabled  IVariant=InternalParameters  DVariant=InternalParameters  IntegratorVariant=Continuous  SatVariant=Disabled  AWVariant=Passthrough  PCopyVariant=Disabled  TRVariant=Disabled  FdbkBlocksVariant=Forward  IdealPFdbkVariant=Disabled  SatFdbkVariant=Disabled  DerivativeFilterVariant=ContFilter  NVariant=InternalParameters  NCopyVariant=Disabled  FilterICVariant=InternalICsFilter  IntegratorICVariant=InternalICs  ExternalResetVariant=Disabled  TRSumVariant=Passthrough  SumFdbkVariant=Disabled  SumVariant=Sum_PID  TsampFilterVariant=InternalTs  TsampNgainVariant=Passthrough  TsampIntegralVariant=Disabled_SignalSpec  ExternalSaturationOutDataTypeStr=Inherit: Same as second input  DerivativeSourceVariant=ErrorSignal  PreIntVariant=InternalPreInt
  Saturation : Saturate  UpperLimit=Tmax  LowerLimit=0
  Sum : Sum  Inputs=|+-
  CMD_TC_delta : Outport
  wires:
  Constant/1 -> Sum/1
  Sum/1 -> PID Controller/1
  PID Controller/1 -> Saturation/1
  kappa_max/1 -> Sum/2
  Saturation/1 -> CMD_TC_delta/1

== system cbuildv0p5/Controls/Traction Control Algorithm/Low Level TC/Torque Reduction Algorithm/Torque Ratio Calculations ==
  CMD_TV_RL : Inport
  CMD_TV_RR : Inport  Port=2
  Divide : Product  Inputs=*/
  Divide1 : Product  Inputs=*/
  Saturation : Saturate  UpperLimit=inf  LowerLimit=0.001
  Sum : Sum  Inputs=|++
  CMD_TV_ratio_RL : Outport
  CMD_TV_ratio_RR : Outport  Port=2
  wires:
  CMD_TV_RL/1 -> Divide/1, Sum/1
  CMD_TV_RR/1 -> Sum/2, Divide1/1
  Sum/1 -> Saturation/1
  Saturation/1 -> Divide1/2, Divide/2
  Divide/1 -> CMD_TV_ratio_RL/1
  Divide1/1 -> CMD_TV_ratio_RR/1

== system cbuildv0p5/Controls/Torque Vectoring/Torque Vectoring Algorithm/Torque Distribution Center/Torque Request Doesn't Surpass T_max/+M_yaw ==
  CMD_TV_delta : Inport
  CMD_T : Inport  Port=2
  Enable : EnablePort  StatesWhenEnabling=reset
  Add : Sum
  Gain : Gain  Gain=0.5
  Subtract : Sum  Inputs=+-
  CMD_TV_RL : Outport
  CMD_TV_RR : Outport  Port=2
  wires:
  CMD_TV_delta/1 -> Gain/1
  Gain/1 -> Add/2, Subtract/2
  CMD_T/1 -> Subtract/1, Add/1
  Subtract/1 -> CMD_TV_RL/1
  Add/1 -> CMD_TV_RR/1

== system cbuildv0p5/Controls/Torque Vectoring/Torque Vectoring Algorithm/Torque Distribution Center/Torque Request Doesn't Surpass T_max/-M_yaw ==
  CMD_TV_delta : Inport
  CMD_T : Inport  Port=2
  Enable : EnablePort  StatesWhenEnabling=reset
  Add : Sum
  Gain : Gain  Gain=0.5
  Subtract : Sum  Inputs=+-
  CMD_TV_RL : Outport
  CMD_TV_RR : Outport  Port=2
  wires:
  CMD_T/1 -> Subtract/1, Add/1
  CMD_TV_delta/1 -> Gain/1
  Gain/1 -> Add/2, Subtract/2
  Subtract/1 -> CMD_TV_RR/1
  Add/1 -> CMD_TV_RL/1

== system cbuildv0p5/Controls/Torque Vectoring/Torque Vectoring Algorithm/Torque Distribution Center/Torque Request Surpasses T_max/+M_yaw ==
  CMD_TV_delta : Inport
  CMD_T : Inport  Port=2
  Enable : EnablePort  StatesWhenEnabling=reset
  Constant : Constant  Value=Tmax
  Subtract : Sum  Inputs=+-
  Subtract1 : Sum  Inputs=+-
  Subtract2 : Sum  Inputs=-+
  CMD_TV_RL : Outport
  CMD_TV_RR : Outport  Port=2
  wires:
  Constant/1 -> CMD_TV_RR/1, Subtract/1
  CMD_TV_delta/1 -> Subtract1/1
  CMD_T/1 -> Subtract2/2, Subtract/2
  Subtract/1 -> Subtract1/2
  Subtract1/1 -> Subtract2/1
  Subtract2/1 -> CMD_TV_RL/1

== system cbuildv0p5/Controls/Torque Vectoring/Torque Vectoring Algorithm/Torque Distribution Center/Torque Request Surpasses T_max/-M_yaw ==
  CMD_TV_delta : Inport
  CMD_T : Inport  Port=2
  Enable : EnablePort  StatesWhenEnabling=reset
  Constant : Constant  Value=Tmax
  Subtract : Sum  Inputs=+-
  Subtract1 : Sum  Inputs=+-
  Subtract2 : Sum  Inputs=-+
  CMD_TV_RL : Outport
  CMD_TV_RR : Outport  Port=2
  wires:
  CMD_T/1 -> Subtract2/2, Subtract/2
  Constant/1 -> CMD_TV_RL/1, Subtract/1
  Subtract/1 -> Subtract1/2
  Subtract1/1 -> Subtract2/1
  CMD_TV_delta/1 -> Subtract1/1
  Subtract2/1 -> CMD_TV_RR/1
